simulink model "AlvaroGaona_08a"  (R2025b)
settings: Solver=VariableStepAuto  StartTime=0.0  StopTime=10  RelTol=1e-3
InitFcn:
  | numero = 8;
  | rng(numero);
  | valor = rand;
  | 
  | M = 1 + valor/2;
  | m = 0.2 * (1 + valor);
  | b = 0.1 * (1 + valor);
  | l = 0.3 * (1.5 - valor/2);
  | g = 9.81;
  | 
  | A = [0, 1, 0, 0;
  | 0, -b/M, -m*g/M, 0;
  | 0, 0, 0, 1;
  | 0, b/(M*l), (M+m)*g/(M*l), 0];
  | 
  | B_ss = [0; 1/M; 0; -1/(M*l)];
  | C_ss = eye(4);
  | D_ss = zeros(4,1);
  | 
  | T = 0.02;
  | sys_d = c2d(ss(A, B_ss, C_ss, D_ss), T, 'zoh');
  | Ad = sys_d.A;
  | Bd = sys_d.B;
  | 
  | % Q = diag([100, 80, 10, 1]);
  | Q = diag([100, 1, 1000, 100]);
  | R = 30;
  | [K, ~, ~] = dlqr(Ad, Bd, Q, R);
  | 
  | x0 = [0; 0; 0.15; 0];
  | X_F = [0.5; 0; 0; 0];
undefined symbols (not defined in the file or in its folder): K
settings Model: Creator=alvaro  LastModifiedBy=alvaro

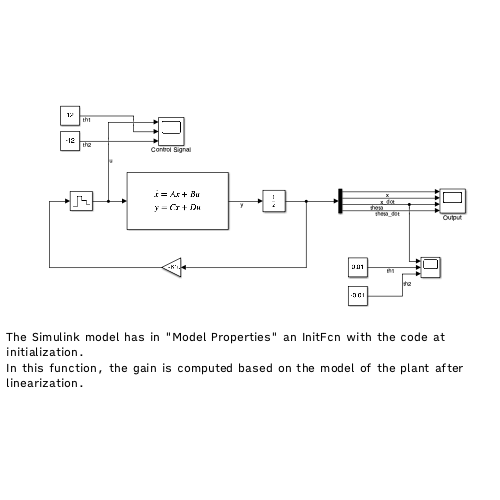
[thumbnail: Simulink's stored preview of the top-level diagram]
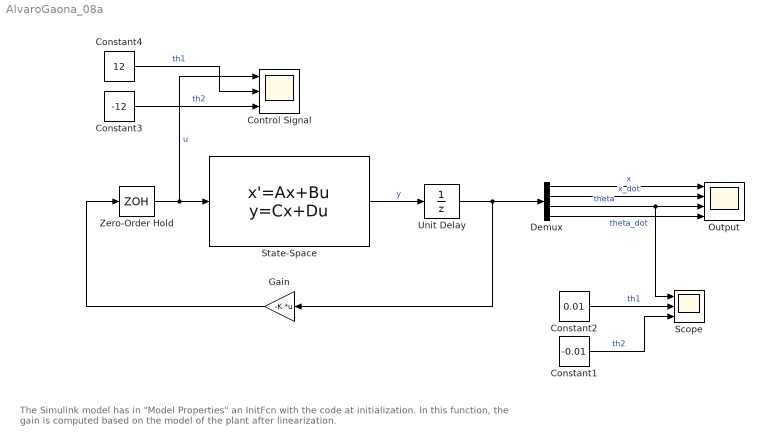
== system AlvaroGaona_08a ==
  note: The Simulink model has in "Model Properties" an InitFcn with the code at initialization.
      | In this function, the gain is computed based on the model of the plant after linearization.
  Constant1 : Constant  Value=-0.01
  Constant2 : Constant  Value=0.01
  Constant3 : Constant  Value=-12
  Constant4 : Constant  Value=12
  Control Signal : Scope  NumInputPorts=3
      settings: ActiveDisplayYMinimum=-15  ActiveDisplayYMaximum=15  DataLoggingVariableName=ScopeData2
  Demux : Demux
  Gain : Gain  Gain=-K  Multiplication=Matrix(K*u)
  Output : Scope  NumInputPorts=4
      settings: ActiveDisplayYMinimum=-0.72019506001372158  ActiveDisplayYMaximum=0.507514129833055
  Scope : Scope  NumInputPorts=3
      settings: ActiveDisplayYMinimum=-0.057855833163501937  ActiveDisplayYMaximum=0.17309509257372241
  State-Space : StateSpace  A=A  B=B_ss  C=C_ss  D=D_ss  InitialCondition=x0
  Unit Delay : UnitDelay  InitialCondition=x0  SampleTime=T  HasFrameUpgradeWarning=on
  Zero-Order Hold : ZeroOrderHold  SampleTime=T
  wires:
  State-Space/1 -> Unit Delay/1  "y"
  Zero-Order Hold/1 -> Control Signal/1, State-Space/1  "u"
  Gain/1 -> Zero-Order Hold/1
  Demux/1 -> Output/1  "x"
  Demux/2 -> Output/2  "x_dot"
  Demux/3 -> Scope/1, Output/3  "theta"
  Demux/4 -> Output/4  "theta_dot"
  Unit Delay/1 -> Gain/1, Demux/1
  Constant2/1 -> Scope/2  "th1"
  Constant1/1 -> Scope/3  "th2"
  Constant4/1 -> Control Signal/2  "th1"
  Constant3/1 -> Control Signal/3  "th2"
